simulink model "min_max_12"  (R2021a)
settings: Solver=VariableStepAuto  StartTime=0.0  StopTime=10.0  RelTol=1e-3
settings Model: Creator=yasso  LastModifiedBy=yasso

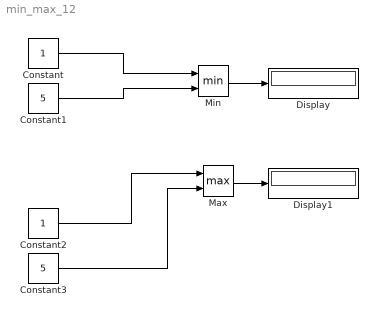
== system min_max_12 ==
  Constant : Constant
  Constant1 : Constant  Value=5
  Constant2 : Constant
  Constant3 : Constant  Value=5
  Display : Display
  Display1 : Display
  Max : MinMax  Function=max  Inputs=2
  Min : MinMax  Inputs=2
  wires:
  Constant/1 -> Min/1
  Constant1/1 -> Min/2
  Constant2/1 -> Max/1
  Constant3/1 -> Max/2
  Min/1 -> Display/1
  Max/1 -> Display1/1
